simulink model "speedEstimatorDirect"  (R2024b)
settings: Solver=FixedStepAuto  StartTime=0.0  StopTime=Tend  FixedStep=Ts  RelTol=1e-3
values from neighbouring files (symbols this model uses):
  Ts = 1e-4    (= 0.0001)    [setup.m]    (also in test.m = 0.001)
undefined symbols (not defined in the file or in its folder): direct
settings Model: Creator=mhmok  LastModifiedBy=mhmok

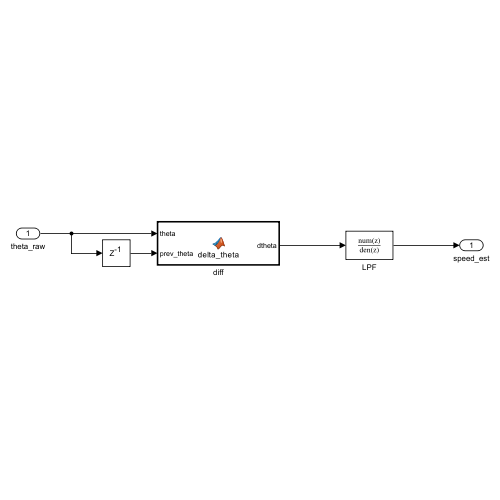
[thumbnail: Simulink's stored preview of the top-level diagram]
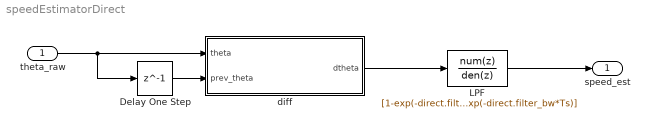
== system speedEstimatorDirect ==
  theta_raw : Inport
  Delay One Step : Delay  DelayLength=1
  LPF : DiscreteTransferFcn  Numerator=[1-exp(-direct.filter_bw*Ts) 0]  Denominator=[1 -exp(-direct.filter_bw*Ts)]
  diff : MATLAB Function  TreatAsAtomicUnit=on
  speed_est : Outport
  wires:
  Delay One Step/1 -> diff/2(prev_theta)
  theta_raw/1 -> Delay One Step/1, diff/1(theta)
  diff/1(dtheta) -> LPF/1
  LPF/1 -> speed_est/1

== matlab function speedEstimatorDirect/diff ==
  data: theta input; dtheta output; prev_theta input; Ts parameter
function dtheta = delta_theta(theta, prev_theta, Ts)

    % check if prev_theta exist before using to prevent error in 1st iteration 
    dtheta = theta - prev_theta;

    % prevent jumps in speed during 2pi to 0 transitions 
    while dtheta > pi
        dtheta = dtheta - 2*pi;
    end

    while dtheta < -pi
        dtheta = dtheta + 2*pi;
    end

    dtheta = dtheta / Ts;
    
end
